simulink model "tcp_node"  (R2019a)
settings: Solver=FixedStepAuto  StartTime=0.0  StopTime=10.0  RelTol=1e-3
libraries: robotlib x1
settings Model: Creator=adeye  LastModifiedBy=adeye
settings OptimizationCC: DefaultParameterBehavior=Inlined  EnhancedBackFolding=on  PassReuseOutputArgsThreshold=0  MaxStackSize=64  OptimizeBlockOrder=speed  DifferentSizesBufferReuse=on  OptimizationCustomize=off
settings DebuggingCC: ParameterTunabilityLossMsg=error
settings HardwareCC: ProdBitPerPointer=32  ProdBitPerSizeT=32  ProdBitPerPtrDiffT=32  ProdLargestAtomicFloat=None  ProdIntDivRoundTo=Undefined  ProdEndianess=Unspecified  ProdWordSize=32  ProdHWDeviceType=Generic->Unspecified (assume 32-bit Generic)  UseEmbeddedCoderFeatures=off
settings SFSimCC: MATLABDynamicMemAlloc=off
settings RTWCC: Description=Generic Real-Time Target  GenerateReport=on  Toolchain=Catkin  LaunchReport=on
settings CodeAppCC: ForceParamTrailComments=on  OperatorAnnotations=on
settings GRTTargetCC: TargetLangStandard=C89/C90 (ANSI)

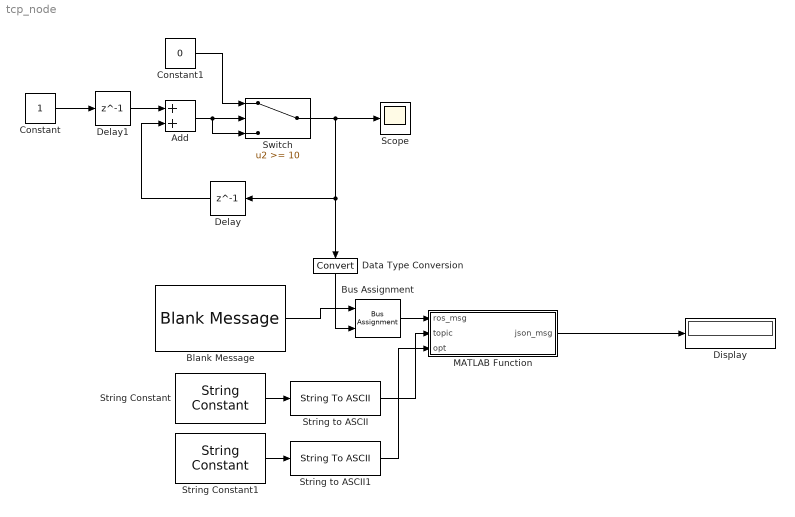
== system tcp_node ==
  Add : Sum
  Blank Message : robotlib/Blank Message  messageClass=Message  entityType=std_msgs/UInt8  messageType=std_msgs/UInt8  SampleTime=inf
      settings: SourceProductBaseCode=RO
  Bus Assignment : BusAssignment  AssignedSignals=Data
  Constant : Constant
  Constant1 : Constant  Value=0
  Data Type Conversion : DataTypeConversion
  Delay : Delay  DelayLength=1
  Delay1 : Delay  DelayLength=1
  Display : Display
  MATLAB Function : MATLAB Function  TreatAsAtomicUnit=on
  Scope : Scope
  String Constant : StringConstant  String="\"/counter\""
  String Constant1 : StringConstant  String="\"publish\""
  String to ASCII : StringToASCII
  String to ASCII1 : StringToASCII
  Switch : Switch  Threshold=10
  wires:
  Blank Message/1 -> Bus Assignment/1
  Data Type Conversion/1 -> Bus Assignment/2
  Constant/1 -> Delay1/1
  Constant1/1 -> Switch/1
  Add/1 -> Switch/3, Switch/2
  Switch/1 -> Delay/1, Data Type Conversion/1, Scope/1
  Delay/1 -> Add/2
  Delay1/1 -> Add/1
  Bus Assignment/1 -> MATLAB Function/1(ros_msg)
  String Constant/1 -> String to ASCII/1
  String to ASCII/1 -> MATLAB Function/2(topic)
  String Constant1/1 -> String to ASCII1/1
  String to ASCII1/1 -> MATLAB Function/3(opt)
  MATLAB Function/1(json_msg) -> Display/1

== matlab function tcp_node/MATLAB Function ==
  data: ros_msg input; topic input; opt input; json_msg output
function json_msg = fcn(ros_msg, topic, opt)

coder.extrinsic('jsonencode');
new_msg = ros_msg;
new_msg.opt = char(opt(opt ~= 0));
new_msg.topic = char(topic(topic ~= 0));
disp(jsonencode(new_msg))
json_msg = 1;
